simulink subsystem "ThreeAxesSignals_magneto"  (R2021a)
settings: Solver=VariableStepAuto  StartTime=0.0  StopTime=10.0  RelTol=1e-3
undefined symbols (not defined in the file): t0x, tfx, wx
libraries: simulink x2
settings Model: Creator=Laura  LastModifiedBy=Laura

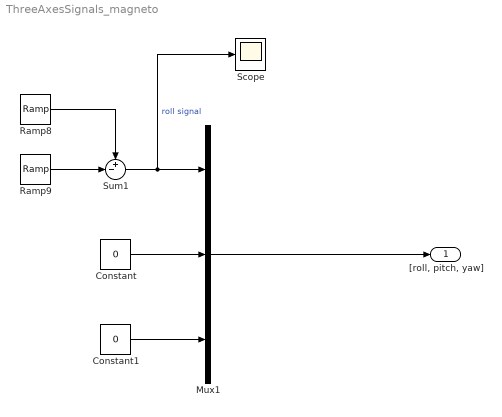
== system ThreeAxesSignals_magneto ==
  Constant : Constant  Value=0
  Constant1 : Constant  Value=0
  Mux1 : Mux  Inputs=3
  Ramp8 : simulink/Sources/Ramp  slope=wx/(tfx - t0x)  start=t0x  InitialOutput=0
  Ramp9 : simulink/Sources/Ramp  slope=wx/(tfx - t0x)  start=tfx  InitialOutput=0
  Scope : Scope
  Sum1 : Sum  Inputs=+-|
  "[roll, pitch, yaw]" : Outport
  wires:
  Mux1/1 -> "[roll, pitch, yaw]"/1
  Ramp9/1 -> Sum1/2
  Ramp8/1 -> Sum1/1
  Sum1/1 -> Scope/1, Mux1/1  "roll signal"
  Constant/1 -> Mux1/2
  Constant1/1 -> Mux1/3
